simulink model "cxema_yst"  (R2015b)
settings: Solver=VariableStepAuto  StartTime=0.0  StopTime=50  RelTol=1e-3
settings Model: Creator=hohotulca  LastModifiedBy=hohotulca

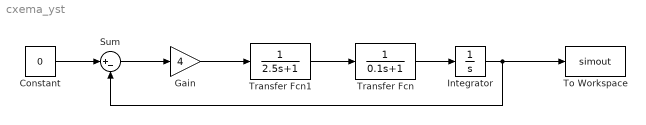
== system cxema_yst ==
  Constant : Constant  Value=0
  Gain : Gain  Gain=4
  Integrator : Integrator  InitialCondition=1
  Sum : Sum  Inputs=|+-
  To Workspace : ToWorkspace  VariableName=simout  SaveFormat=Timeseries  SampleTime=-1
  Transfer Fcn : TransferFcn  Denominator=[0.1 1]
  Transfer Fcn1 : TransferFcn  Denominator=[2.5 1]
  wires:
  Transfer Fcn/1 -> Integrator/1
  Sum/1 -> Gain/1
  Gain/1 -> Transfer Fcn1/1
  Transfer Fcn1/1 -> Transfer Fcn/1
  Integrator/1 -> To Workspace/1, Sum/2
  Constant/1 -> Sum/1
